simulink model "sm_motor_grader_FrameF"  (R2025a)
settings: Solver=daessc  StartTime=0.0  StopTime=stopTime  MaxStep=0.01  RelTol=1e-3  EnableMultiTasking=on
PostLoadFcn:
  | warning off SimulinkBlock:Foundation:RuntimeAccessInvalidSource
undefined symbols (not defined in the file): motGradParams, X, Y, Z
libraries: sm_motor_grader_lib x16, sm_lib x4, nesl_utility x1
Description:
  | Copyright 2025 The MathWorks, Inc.
settings Model: Creator=smiller  LastModifiedBy=smiller
settings SolverCC: AlgebraicLoopSolver=TrustRegion  MaxZcPerStep=1.0
settings DataIOCC: LimitDataPoints=on  MaxDataPoints=10000  ReturnWorkspaceOutputs=off  SignalLoggingName=logsout_sm_motor_grader_FrameF
settings OptimizationCC: ReuseModelBlockBuffer=off  LifeSpan=inf
settings DebuggingCC: UnconnectedInputMsg=warning  UnconnectedOutputMsg=warning  UnconnectedLineMsg=warning  AllowSymbolicDim=off  SubsystemReferenceDiagnosticForUnitTest=warning  SFUnexpectedBacktrackingDiag=warning  SFNoUnconditionalDefaultTransitionDiag=warning  SFExecutionAtInitializationDiag=none  ArithmeticOperatorsInVariantConditions=warning
settings ModelReferenceCC: EnableRefExpFcnMdlSchedulingChecks=on
settings SFSimCC: SimUseLocalCustomCode=off  CustomCodeUndefinedFunction=UseInterfaceOnly
settings RTWCC: RTWUseLocalCustomCode=off  GPUComputeCapability=3.5  DLArmComputeVersion=19.05
settings CodeAppCC: StateflowObjectComments=on
settings GRTTargetCC: TargetLangStandard=C89/C90 (ANSI)
settings ConfigComp: CovMetricSettings=dw  CovSaveCumulativeToWorkspaceVar=on  CovSaveSingleToWorkspaceVar=on  CovExternalEMLEnable=off  CovSFcnEnable=off
settings SimscapeCC: SimscapeLogType=all  SimscapeLogSimulationStatistics=on  SimscapeLogName=simlog_sm_motor_grader_FrameF  SimscapeLogDataHistory=10000.0
settings ExplorerConfigSet: InternalSimMechanicsExplorerSettings="<ExplorerConfiguration><canonicalview>default</canonicalview><AnimationSetting><BasePlaybackSpeed>1.0</BasePlaybackSpeed><PlaybackSpeedFactor>4.0</PlaybackSpeedFactor></AnimationSetting><TilePanel><TileInfo><Tiles Columns=\"1\" Count=\"1\" Rows=\"1\"><Column Weight=\"1\"/><Row Weight=\"1\"/><Tile Height=\"1\" Width=\"1\" X=\"0\" Y=\"0\"/></Tiles></TileInfo><SceneInfo><SceneViewer><BGColor><R>1</R><G>1</G><B>1</B></BGColor><Camera><DoPerspective>off</DoPerspective><Position><X>-2.76363722089077113</X><Y>-0.296535843489885598</Y><Z>1.12928046769726942</Z></Position><Center><X>-0.0232155150432307167</X><Y>0.0238804081777167498</Y><Z>0.906060622936961213</Z></Center><Up><X>0.081843009395675681</X><Y>-0.0056706428820125776</Y><Z>0.996629101332268341</Z></Up><ViewLimDist>1</ViewLimDist><YLim>1.48175750570382903</YLim><XLim>2.01181710124015822</XLim></Camera></SceneViewer></SceneInfo></TilePanel><MechEditorPanel><Cameras/><GfxPanelCameraMap/><VideoCreator><PlaybackSpeedRatio>1.0</PlaybackSpeedRatio><FrameRate>30</FrameRate><VideoFormat>Motion JPEG AVI</VideoFormat><FrameSize>auto</FrameSize></VideoCreator></MechEditorPanel></ExplorerConfiguration>"

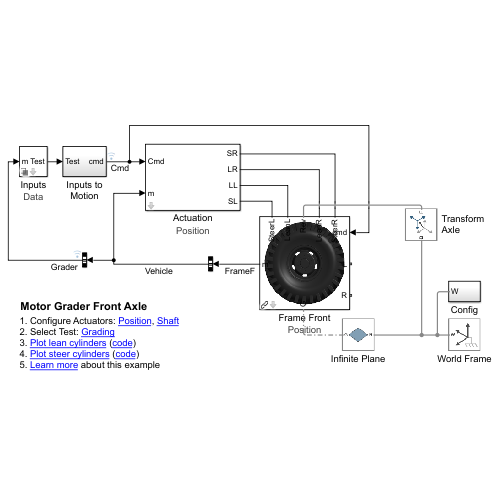
[thumbnail: Simulink's stored preview of the top-level diagram]
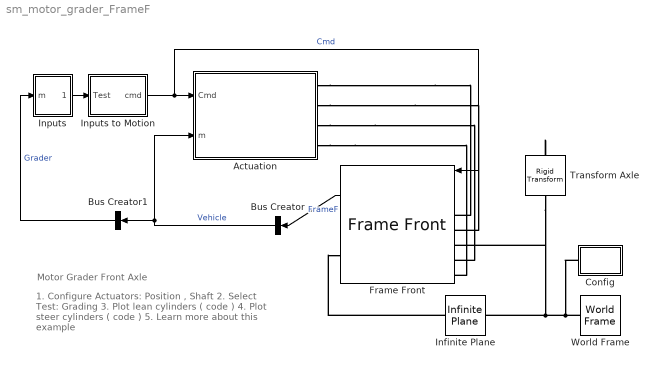
== system sm_motor_grader_FrameF ==
  note: 1. Configure Actuators: Position , Shaft
      | 2. Select Test: Grading
      | 3. Plot lean cylinders ( code )
      | 4. Plot steer cylinders ( code )
      | 5. Learn more about this example
  note: Motor Grader Front Axle
  Actuation : Subsystem  VariantControl=Actuation  mask{popup_actuator_model=Position}
      mask prompts: popup_actuator_model "Actuation Mode"
      mask init:
      | bh = gcb;
      | modestr = get_param(bh,'popup_actuator_model');
      | set_param([bh '/Actuator SteerL'],'LabelModeActiveChoice',modestr)
      | set_param([bh '/Actuator SteerR'],'LabelModeActiveChoice',modestr)
      | set_param([bh '/Actuator LeanL'],'LabelModeActiveChoice',modestr)
      | set_param([bh '/Actuator LeanR'],'LabelModeActiveChoice',modestr)
      settings: AttributesFormatString=%<popup_actuator_model>
      mask TypeOptions popup_actuator_model: Position | Shaft
  Bus Creator : BusCreator  Inputs=1
  Bus Creator1 : BusCreator  Inputs=1
  Config : Subsystem
  Frame Front : sm_motor_grader_lib/Frame Front  popup_actuator_model=Position  popup_ground_contact=Sphere
      settings: AttributesFormatString=%<popup_actuator_model>
  Infinite Plane : sm_lib/Curves and Surfaces/Infinite Plane  GraphicType=Rectangle  GraphicPlaneWidth=2  GraphicPlaneWidthUnits=m  GraphicPlaneHeight=4  GraphicPlaneHeightUnits=m  GraphicVisPropType=SimpleVisualProperties  GraphicDiffuseColor=[0.5 0.5 0.5]  GraphicOpacity=0.5  GraphicSpecularColor=[0.5 0.5 0.5 1.0]  GraphicAmbientColor=[0.15 0.15 0.15 1.0]  GraphicEmissiveColor=[0.0 0.0 0.0 1.0]  GraphicShininess=75
  Inputs : Subsystem  Variant=on  VariantControlMode=label  VariantControl=Inputs  LabelModeActiveChoice=Data  mask{test_source=Data}
      mask prompts: test_source "Test Source"
      mask init:
      | bh = gcb;
      | data_source = get_param(bh,'test_source');
      | set_param(bh,'LabelModeActiveChoice',data_source)
      settings: AttributesFormatString=%<LabelModeActiveChoice>
      mask TypeOptions test_source: Data | Dashboard
      mask Display: disp(' ')
  Inputs to Motion : Subsystem
  Transform Axle : sm_lib/Frames and Transforms/Rigid Transform  RotationMethod=RotationSequence  FollAlignAxisA=+X  BaseAlignAxisA=+Y  FollAlignAxisB=+Y  BaseAlignAxisB=+Z  RotationStandardAxis=+X  RotationAngle=-90  RotationAngleUnits=deg  RotationArbitraryAxis=[0 0 1]  RotationSequenceAxes=FollowerAxes  RotationSequence=XYX  RotationSequenceAngles=[-90 90 0]  RotationSequenceAnglesUnits=deg  RotationMatrix=[1 0 0;0 1 0;0 0 1]  Quaternion=[1 0 0 0]  TranslationMethod=StandardAxis  TranslationCartesianOffset=[0 0 0]  TranslationCartesianOffsetUnits=m  TranslationStandardAxis=+Z  TranslationStandardOffset=motGradParams.groundContact.tireRad+0.08  TranslationStandardOffsetUnits=m  TranslationROffset=0  TranslationROffsetUnits=m  TranslationThetaOffset=0  TranslationThetaOffsetUnits=deg  TranslationZOffset=0  TranslationZOffsetUnits=m
  World Frame : sm_lib/Frames and Transforms/World Frame
  wires:
  Inputs/1(Test) -> Inputs to Motion/1(Test)
  Inputs to Motion/1(cmd) -> Frame Front/1, Actuation/1(Cmd)  "Cmd"
  Frame Front/1 -> Bus Creator/1  "FrameF"
  Bus Creator/1 -> Actuation/2(m), Bus Creator1/1  "Vehicle"
  Bus Creator1/1 -> Inputs/1(m)  "Grader"
  connections:
  World Frame/RConn1 -- Transform Axle/LConn1 -- Infinite Plane/LConn1 -- Config/LConn1
  Actuation/RConn4 -- Frame Front/LConn7
  Actuation/RConn1 -- Frame Front/LConn3
  Actuation/RConn3 -- Frame Front/LConn6
  Actuation/RConn2 -- Frame Front/LConn4
  Infinite Plane/RConn1 -- Frame Front/RConn1
  Transform Axle/RConn1 -- Frame Front/LConn5

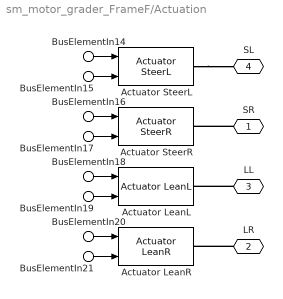
== system sm_motor_grader_FrameF/Actuation ==
  BusElementIn14 : Inport  PortName=Cmd  Element=pSteerL
  BusElementIn16 : Inport  PortName=Cmd  Element=pSteerR
  BusElementIn18 : Inport  PortName=Cmd  Element=pLeanL
  BusElementIn20 : Inport  PortName=Cmd  Element=pLeanR
  BusElementIn15 : Inport  Port=2  PortName=m  Element=FrameF.SteerL.p
  BusElementIn17 : Inport  Port=2  PortName=m  Element=FrameF.SteerR.p
  BusElementIn19 : Inport  Port=2  PortName=m  Element=FrameF.LeanL.p
  BusElementIn21 : Inport  Port=2  PortName=m  Element=FrameF.LeanR.p
  Actuator LeanL : sm_motor_grader_lib/Actuation/Actuator LeanL  SystemSampleTime=-1  VariantControl=Actuator LeanL  LabelModeActiveChoice=Position  VariantActivationTime=update diagram  EmptyChoice=off  PassThrough=off  PassThroughVariantControl=(default)  EmptyChoiceVariantControl=(default)  AllowFlexibleInterface=on  Latency=0  AutoFrameSizeCalculation=off
  Actuator LeanR : sm_motor_grader_lib/Actuation/Actuator LeanR  SystemSampleTime=-1  VariantControl=Actuator LeanR  LabelModeActiveChoice=Position  VariantActivationTime=update diagram  EmptyChoice=off  PassThrough=off  PassThroughVariantControl=(default)  EmptyChoiceVariantControl=(default)  AllowFlexibleInterface=on  Latency=0  AutoFrameSizeCalculation=off
  Actuator SteerL : sm_motor_grader_lib/Actuation/Actuator SteerL  SystemSampleTime=-1  VariantControl=Actuator SteerL  LabelModeActiveChoice=Position  VariantActivationTime=update diagram  EmptyChoice=off  PassThrough=off  PassThroughVariantControl=(default)  EmptyChoiceVariantControl=(default)  AllowFlexibleInterface=on  Latency=0  AutoFrameSizeCalculation=off
  Actuator SteerR : sm_motor_grader_lib/Actuation/Actuator SteerR  SystemSampleTime=-1  VariantControl=Actuator SteerR  LabelModeActiveChoice=Position  VariantActivationTime=update diagram  EmptyChoice=off  PassThrough=off  PassThroughVariantControl=(default)  EmptyChoiceVariantControl=(default)  AllowFlexibleInterface=on  Latency=0  AutoFrameSizeCalculation=off
  SR : PMIOPort  Side=Right
  LR : PMIOPort  Port=2  Side=Right
  LL : PMIOPort  Port=3  Side=Right
  SL : PMIOPort  Port=4  Side=Right
  wires:
  BusElementIn14/1 -> Actuator SteerL/1
  BusElementIn15/1 -> Actuator SteerL/2
  BusElementIn16/1 -> Actuator SteerR/1
  BusElementIn17/1 -> Actuator SteerR/2
  BusElementIn20/1 -> Actuator LeanR/1
  BusElementIn21/1 -> Actuator LeanR/2
  BusElementIn19/1 -> Actuator LeanL/2
  BusElementIn18/1 -> Actuator LeanL/1
  connections:
  Actuator SteerL/RConn1 -- SL/RConn1
  SR/RConn1 -- Actuator SteerR/RConn1
  LL/RConn1 -- Actuator LeanL/RConn1
  LR/RConn1 -- Actuator LeanR/RConn1

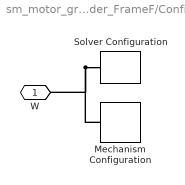
== system sm_motor_grader_FrameF/Config ==
  Mechanism Configuration : sm_lib/Utilities/Mechanism Configuration  UniformGravity=Constant  GravityVector=[0 0 -9.80665]  GravityVectorUnits=m/s^2  LinearizationDelta=0.001  JointModeTransitionNonlinearIterations=2
  Solver Configuration : nesl_utility/Solver Configuration  PhysicalDomain=network_engine_domain  SubClassName=solver  LeftPortType=input  RightPortType=generic  Tones=[]  Harmonics=[]  SimulateNoise=off  Profile=off  UseLocalSampling=off  EnableSwitchedLinearOptims=on  FrequencyDomain=off  UseCCode=off  RelTol=0.001  AbsTol=1e-06  MinStep=1e-09  ToWorkspace=off  RevertToSquareIcSolve=off  NumHomotopyIterations=100  PhasorMode=off  PhasorModeNumHarmonics=1  ConsistencySolver=NEWTON_XTOL_AFTER_FTOL  IndexReductionMethod=DerivativeReplacement  DoDC=off  ResidualTolerance=1e-09  ConsistencyTolSource=GLOBAL  ConsistencyAbsTol=0.001  ConsistencyRelTol=0.001  ConsistencyTolFactor=0.001  UseLocalSolver=off  LocalSolverChoice=NE_BACKWARD_EULER_ADVANCER  ResolveIndetEquations=on  FunctionEvalNumThread=1  LocalSolverSampleTime=0.001  DoFixedCost=off  MaxNonlinIter=3  MaxModeIter=2  ComputeImpulses=off  ImpulseIterations=2  LinearAlgebra=Sparse  LinearAlgebraNumThread=0  EquationFormulation=NE_TIME_EF  DelaysMemoryBudget=1024  AutomaticFiltering=on  FilteringTimeConstant=0.001  PartitionStorageMethod=AS_NEEDED  PartitionMemoryBudget=1024  PartitionMethod=FAST  MultibodyUseLocalSolver=off  MultibodyLocalSolverChoice=ODE1  MultibodyLocalSolverSampleTime=0.001
  W : PMIOPort  Side=Left
  connections:
  Solver Configuration/RConn1 -- Mechanism Configuration/RConn1 -- W/RConn1

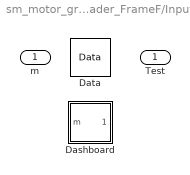
== system sm_motor_grader_FrameF/Inputs ==
  m : Inport
  Dashboard : Subsystem  VariantControl=Dashboard
  Data : sm_motor_grader_lib/Data  SystemSampleTime=-1  VariantControl=Data  VariantActivationTime=update diagram  EmptyChoice=off  PassThrough=off  PassThroughVariantControl=(default)  EmptyChoiceVariantControl=(default)  AllowFlexibleInterface=on  Latency=0  AutoFrameSizeCalculation=off
  Test : Outport

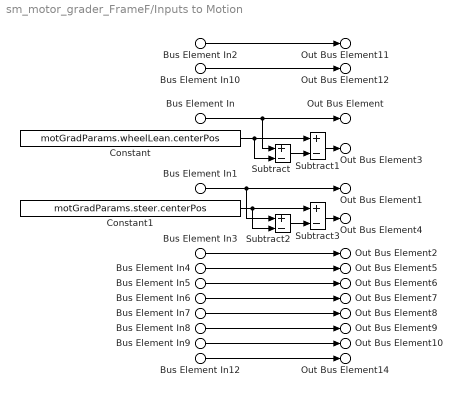
== system sm_motor_grader_FrameF/Inputs to Motion ==
  Bus Element In : Inport  PortName=Test  Element=pLean
  Bus Element In1 : Inport  PortName=Test  Element=pSteer
  Bus Element In2 : Inport  PortName=Test  Element=vVeh
  Bus Element In3 : Inport  PortName=Test  Element=pArtic
  Bus Element In4 : Inport  PortName=Test  Element=pLiftL
  Bus Element In5 : Inport  PortName=Test  Element=pLiftR
  Bus Element In6 : Inport  PortName=Test  Element=pCircleShift
  Bus Element In7 : Inport  PortName=Test  Element=qCircle
  Bus Element In8 : Inport  PortName=Test  Element=pTilt
  Bus Element In9 : Inport  PortName=Test  Element=pShift
  Bus Element In10 : Inport  PortName=Test  Element=nHoleLink
  Bus Element In12 : Inport  PortName=Test  Element=pPin
  Constant : Constant  Value=motGradParams.wheelLean.centerPos
  Constant1 : Constant  Value=motGradParams.steer.centerPos
  Subtract{,1..3} (4 alike) : Sum  Inputs=+-
  Out Bus Element : Outport  PortName=cmd  Element=pLeanL
  Out Bus Element1 : Outport  PortName=cmd  Element=pSteerL
  Out Bus Element2 : Outport  PortName=cmd  Element=pArtic
  Out Bus Element3 : Outport  PortName=cmd  Element=pLeanR
  Out Bus Element4 : Outport  PortName=cmd  Element=pSteerR
  Out Bus Element5 : Outport  PortName=cmd  Element=pLiftL
  Out Bus Element6 : Outport  PortName=cmd  Element=pLiftR
  Out Bus Element7 : Outport  PortName=cmd  Element=pCircleShift
  Out Bus Element8 : Outport  PortName=cmd  Element=qCircle
  Out Bus Element9 : Outport  PortName=cmd  Element=pTilt
  Out Bus Element10 : Outport  PortName=cmd  Element=pShift
  Out Bus Element11 : Outport  PortName=cmd  Element=vVeh
  Out Bus Element12 : Outport  PortName=cmd  Element=nHoleLink
  Out Bus Element14 : Outport  PortName=cmd  Element=pPin
  wires:
  Bus Element In/1 -> Subtract/1, Out Bus Element/1
  Subtract1/1 -> Out Bus Element3/1
  Subtract3/1 -> Out Bus Element4/1
  Subtract/1 -> Subtract1/2
  Bus Element In1/1 -> Subtract2/1, Out Bus Element1/1
  Constant/1 -> Subtract/2, Subtract1/1
  Subtract2/1 -> Subtract3/2
  Constant1/1 -> Subtract2/2, Subtract3/1
  Bus Element In2/1 -> Out Bus Element11/1
  Bus Element In3/1 -> Out Bus Element2/1
  Bus Element In4/1 -> Out Bus Element5/1
  Bus Element In5/1 -> Out Bus Element6/1
  Bus Element In6/1 -> Out Bus Element7/1
  Bus Element In7/1 -> Out Bus Element8/1
  Bus Element In8/1 -> Out Bus Element9/1
  Bus Element In9/1 -> Out Bus Element10/1
  Bus Element In10/1 -> Out Bus Element12/1
  Bus Element In12/1 -> Out Bus Element14/1

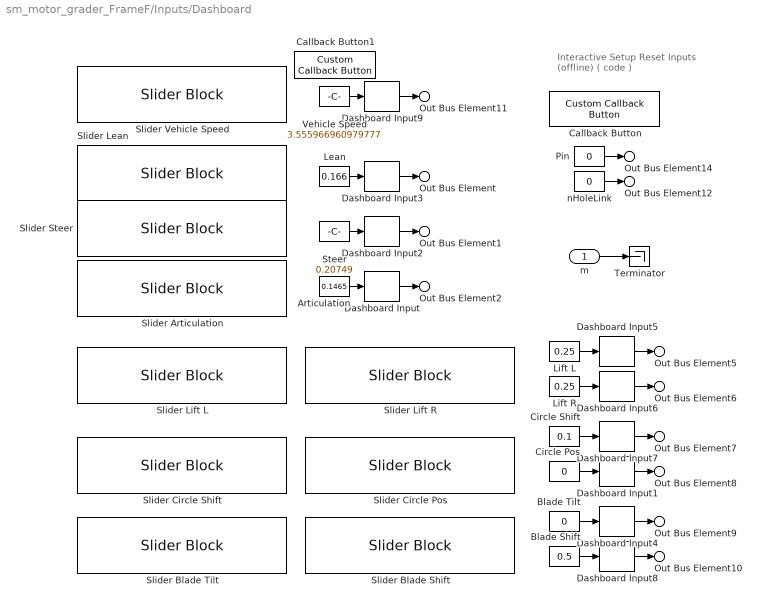
== system sm_motor_grader_FrameF/Inputs/Dashboard ==
  note: Interactive Setup
      | Reset Inputs (offline) ( code )
  m : Inport
  Articulation : Constant  Value=0.1465
  Blade Shift : Constant  Value=0.5
  Blade Tilt : Constant  Value=0
  Callback Button : CustomCallbackButton  Configuration="{\"components\":[{\"name\":\"BackgroundImageComponent\",\"settings\":{\"image\":{\"size\":[0,0],\"src\":\"default\",\"srcOrientation\":\"Right\"},\"position\":[0,0,1,1]}},{\"name\":\"ButtonStateComponent\",\"settings\":{\"buttonType\":\"momentary\",\"clickFcn\":\"sm_motor_grader_init_dashboard_values(gcs,motGradParams)\",\"onValue\":1,\"position\":[0,0,1,1],\"pressDelay\":\"500\",\"pressFcn\":\"\",\"repeatInterval\":\"0\",\"states\":[{\"horizontalAlignment\":\"center\",\"image\":{\"position\":[0,0,1,1],\"size\":[1,1],\"src\":\"default\",\"srcOrientation\":\"Right\"},\"label\":{\"color\":[0.01176470588,0.01176470588,0.01176470588,1],\"icon\":{\"size\":[0,0],\"src\":\"default\",\"srcOrientation\":\"Right\"},\"iconOffset\":0,\"iconPlacement\":\"left\",\"opacity\":1,\"show\":true,\"text\":{\"content\":\"Reset Inputs\",\"font\":\"Arial\"}},\"labelOffset\":[0,0],\"verticalAlignment\":\"middle\"},{\"horizontalAlignment\":\"center\",\"image\":{\"position\":[0,0,1,1],\"size\":[1,1],\"src\":\"default\",\"srcOrientation\":\"Right\"},\"label\":{\"color\":[0.01176470588,0.01176470588,0.01176470588,1],\"icon\":{\"size\":[0,0],\"src\":\"default\",\"srcOrientation\":\"Right\"},\"iconOffset\":0,\"iconPlacement\":\"left\",\"opacity\":1,\"show\":true,\"text\":{\"content\":\"Reset Inputs\",\"font\":\"Arial\"}},\"labelOffset\":[0,0],\"verticalAlignment\":\"middle\"},{\"horizontalAlignment\":\"center\",\"image\":{\"position\":[0,0,1,1],\"size\":[1,1],\"src\":\"default\",\"srcOrientation\":\"Right\"},\"label\":{\"color\":[0.01176470588,0.01176470588,0.01176470588,1],\"icon\":{\"size\":[0,0],\"src\":\"default\",\"srcOrientation\":\"Right\"},\"iconOffset\":0,\"iconPlacement\":\"left\",\"opacity\":1,\"show\":true,\"text\":{\"content\":\"Reset Inputs\",\"font\":\"Arial\"}},\"labelOffset\":[0,0],\"verticalAlignment\":\"middle\"},{\"horizontalAlignment\":\"center\",\"image\":{\"position\":[0,0,1,1],\"size\":[1,1],\"src\":\"default\",\"srcOrientation\":\"Right\"},\"label\":{\"color\":[0.01176470588,0.01176470588,0.01176470588,1],\"icon\":{\"size\":[0,0],\"src\":\"default\",\"srcOrientation\":\"Right\"},\"iconOffset\":0,\"iconPlacement\":\"left\",\"opacity\":1,\"show\":true,\"text\":{\"content\":\"Reset Inputs\",\"font\":\"Arial\"}},\"labelOffset\":[0,0],\"verticalAlignment\":\"middle\"}]}},{\"name\":\"ForegroundImageComponent\",\"settings\":{\"image\":{\"size\":[0,0],\"src\":\"default\",\"srcOrientation\":\"Right\"},\"isForeground\":1,\"position\":[0,0,1,1]}}],\"settings\":{\"BindingType\":\"standalone\",\"backgroundColor\":[244,244,244,1],\"backgroundOffset\":0.2,\"backgroundOpacity\":1,\"fixedAspectRatio\":\"off\",\"foregroundColor\":[0.01176470588,0.01176470588,0.01176470588,1],\"migratedFromLegacy\":true,\"useBackgroundColor\":true,\"variant\":\"callback\",\"version\":\"R2023a\"},\"type\":\"Button\"}"  CustomBackgroundColor="{\"color\":[0.9568627451,0.9568627451,0.9568627451],\"show\":true}"
  Callback Button1 : CustomCallbackButton  Configuration="{\"components\":[{\"name\":\"BackgroundImageComponent\",\"settings\":{\"image\":{\"size\":[0,0],\"src\":\"default\",\"srcOrientation\":\"Right\"},\"position\":[0,0,1,1]}},{\"name\":\"ButtonStateComponent\",\"settings\":{\"buttonType\":\"momentary\",\"clickFcn\":\"set_param([gcs '\\/Vehicle Speed'],'Value','0')\",\"onValue\":1,\"position\":[0,0,1,1],\"pressDelay\":\"500\",\"pressFcn\":\"\",\"repeatInterval\":\"0\",\"states\":[{\"horizontalAlignment\":\"center\",\"image\":{\"position\":[0,0,1,1],\"size\":[1,1],\"src\":\"default\",\"srcOrientation\":\"Right\"},\"label\":{\"color\":[0.01176470588,0.01176470588,0.01176470588,1],\"icon\":{\"size\":[0,0],\"src\":\"default\",\"srcOrientation\":\"Right\"},\"iconOffset\":0,\"iconPlacement\":\"left\",\"opacity\":1,\"show\":true,\"text\":{\"content\":\"Stop Grader\",\"font\":\"Arial\"}},\"labelOffset\":[0,0],\"verticalAlignment\":\"middle\"},{\"horizontalAlignment\":\"center\",\"image\":{\"position\":[0,0,1,1],\"size\":[1,1],\"src\":\"default\",\"srcOrientation\":\"Right\"},\"label\":{\"color\":[0.01176470588,0.01176470588,0.01176470588,1],\"icon\":{\"size\":[0,0],\"src\":\"default\",\"srcOrientation\":\"Right\"},\"iconOffset\":0,\"iconPlacement\":\"left\",\"opacity\":1,\"show\":true,\"text\":{\"content\":\"Stop Grader\",\"font\":\"Arial\"}},\"labelOffset\":[0,0],\"verticalAlignment\":\"middle\"},{\"horizontalAlignment\":\"center\",\"image\":{\"position\":[0,0,1,1],\"size\":[1,1],\"src\":\"default\",\"srcOrientation\":\"Right\"},\"label\":{\"color\":[0.01176470588,0.01176470588,0.01176470588,1],\"icon\":{\"size\":[0,0],\"src\":\"default\",\"srcOrientation\":\"Right\"},\"iconOffset\":0,\"iconPlacement\":\"left\",\"opacity\":1,\"show\":true,\"text\":{\"content\":\"Stop Grader\",\"font\":\"Arial\"}},\"labelOffset\":[0,0],\"verticalAlignment\":\"middle\"},{\"horizontalAlignment\":\"center\",\"image\":{\"position\":[0,0,1,1],\"size\":[1,1],\"src\":\"default\",\"srcOrientation\":\"Right\"},\"label\":{\"color\":[0.01176470588,0.01176470588,0.01176470588,1],\"icon\":{\"size\":[0,0],\"src\":\"default\",\"srcOrientation\":\"Right\"},\"iconOffset\":0,\"iconPlacement\":\"left\",\"opacity\":1,\"show\":true,\"text\":{\"content\":\"Stop Grader\",\"font\":\"Arial\"}},\"labelOffset\":[0,0],\"verticalAlignment\":\"middle\"}]}},{\"name\":\"ForegroundImageComponent\",\"settings\":{\"image\":{\"size\":[0,0],\"src\":\"default\",\"srcOrientation\":\"Right\"},\"isForeground\":1,\"position\":[0,0,1,1]}}],\"settings\":{\"BindingType\":\"standalone\",\"backgroundColor\":[244,244,244,1],\"backgroundOffset\":0.2,\"backgroundOpacity\":1,\"fixedAspectRatio\":\"off\",\"foregroundColor\":[0.01176470588,0.01176470588,0.01176470588,1],\"migratedFromLegacy\":true,\"useBackgroundColor\":true,\"variant\":\"callback\",\"version\":\"R2023a\"},\"type\":\"Button\"}"  CustomBackgroundColor="{\"color\":[0.9568627451,0.9568627451,0.9568627451],\"show\":true}"
  Circle Pos : Constant  Value=0
  Circle Shift : Constant  Value=0.1
  Dashboard Input : sm_motor_grader_lib/Dashboard Input  upper_bound=motGradParams.articulation.upperBound  lower_bound=motGradParams.articulation.lowerBound  U0=motGradParams.articulation.initPos  tfilt=1
  Dashboard Input1 : sm_motor_grader_lib/Dashboard Input  upper_bound=motGradParams.circleRot.maxPos  lower_bound=motGradParams.circleRot.minPos  U0=motGradParams.circleRot.initPos  tfilt=1
  Dashboard Input2 : sm_motor_grader_lib/Dashboard Input  upper_bound=motGradParams.steer.upperBound  lower_bound=motGradParams.steer.lowerBound  U0=motGradParams.steer.initPos  tfilt=1
  Dashboard Input3 : sm_motor_grader_lib/Dashboard Input  upper_bound=motGradParams.wheelLean.upperBound  lower_bound=motGradParams.wheelLean.lowerBound  U0=motGradParams.wheelLean.initPos  tfilt=1
  Dashboard Input4 : sm_motor_grader_lib/Dashboard Input  upper_bound=motGradParams.bladeTilt.stroke  lower_bound=0  U0=motGradParams.bladeTilt.initPos  tfilt=1
  Dashboard Input5 : sm_motor_grader_lib/Dashboard Input  upper_bound=motGradParams.bladeLift.stroke  lower_bound=0  U0=motGradParams.bladeLift.leftInitPos  tfilt=1
  Dashboard Input6 : sm_motor_grader_lib/Dashboard Input  upper_bound=motGradParams.bladeLift.stroke  lower_bound=0  U0=motGradParams.bladeLift.rightInitPos  tfilt=1
  Dashboard Input7 : sm_motor_grader_lib/Dashboard Input  upper_bound=motGradParams.circleShift.stroke  lower_bound=0  U0=motGradParams.circleShift.initPos  tfilt=1
  Dashboard Input8 : sm_motor_grader_lib/Dashboard Input  upper_bound=motGradParams.bladeSideShift.stroke  lower_bound=0  U0=motGradParams.bladeSideShift.initPos  tfilt=1
  Dashboard Input9 : sm_motor_grader_lib/Dashboard Input  upper_bound=motGradParams.drivetrain.topSpeed  lower_bound=-motGradParams.drivetrain.topSpeed  U0=0  tfilt=1
  Lean : Constant  Value=0.166
  Lift L : Constant  Value=0.25
  Lift R : Constant  Value=0.25
  Pin : Constant  Value=0
  Slider Articulation : SliderBlock  ScaleMin=0.076499999999999985  ScaleMax=0.2165
  Slider Blade Shift : SliderBlock  ScaleMax=1.3
  Slider Blade Tilt : SliderBlock  ScaleMax=0.20000000000000001
  Slider Circle Pos : SliderBlock  ScaleMin=-90  ScaleMax=90
  Slider Circle Shift : SliderBlock  ScaleMax=0.84999999999999998
  Slider Lean : SliderBlock  ScaleMin=0.10000000000000001  ScaleMax=0.23200000000000001
  Slider Lift L : SliderBlock  ScaleMax=1.2
  Slider Lift R : SliderBlock  ScaleMax=1.2
  Slider Steer : SliderBlock  ScaleMin=0.14748700000000001  ScaleMax=0.26748700000000003
  Slider Vehicle Speed : SliderBlock  ScaleMin=-11  ScaleMax=11
  Steer : Constant  Value=0.20749
  Terminator : Terminator
  Vehicle Speed : Constant  Value=3.555966960979777
  nHoleLink : Constant  Value=0
  Out Bus Element : Outport  PortName=Test  Element=pLean
  Out Bus Element1 : Outport  PortName=Test  Element=pSteer
  Out Bus Element2 : Outport  PortName=Test  Element=pArtic
  Out Bus Element5 : Outport  PortName=Test  Element=pLiftL
  Out Bus Element6 : Outport  PortName=Test  Element=pLiftR
  Out Bus Element7 : Outport  PortName=Test  Element=pCircleShift
  Out Bus Element8 : Outport  PortName=Test  Element=qCircle
  Out Bus Element9 : Outport  PortName=Test  Element=pTilt
  Out Bus Element10 : Outport  PortName=Test  Element=pShift
  Out Bus Element11 : Outport  PortName=Test  Element=vVeh
  Out Bus Element12 : Outport  PortName=Test  Element=nHoleLink
  Out Bus Element14 : Outport  PortName=Test  Element=pPin
  wires:
  Dashboard Input9/1 -> Out Bus Element11/1
  Vehicle Speed/1 -> Dashboard Input9/1
  Lift L/1 -> Dashboard Input5/1
  Lift R/1 -> Dashboard Input6/1
  Circle Shift/1 -> Dashboard Input7/1
  Circle Pos/1 -> Dashboard Input1/1
  Blade Tilt/1 -> Dashboard Input4/1
  Blade Shift/1 -> Dashboard Input8/1
  Lean/1 -> Dashboard Input3/1
  Steer/1 -> Dashboard Input2/1
  Dashboard Input/1 -> Out Bus Element2/1
  nHoleLink/1 -> Out Bus Element12/1
  Pin/1 -> Out Bus Element14/1
  Articulation/1 -> Dashboard Input/1
  Dashboard Input1/1 -> Out Bus Element8/1
  Dashboard Input2/1 -> Out Bus Element1/1
  Dashboard Input3/1 -> Out Bus Element/1
  Dashboard Input4/1 -> Out Bus Element9/1
  Dashboard Input5/1 -> Out Bus Element5/1
  Dashboard Input6/1 -> Out Bus Element6/1
  Dashboard Input7/1 -> Out Bus Element7/1
  Dashboard Input8/1 -> Out Bus Element10/1
  m/1 -> Terminator/1
